simulink subsystem "Counter"  (R2022b)
settings: Solver=VariableStepAuto  StartTime=0.0  StopTime=10.0  RelTol=1e-3
model mask{counterType=Up, value=1, reset=0, cntValue=1}
  mask prompts: counterType "Counter Type"; value "Counter Value"; reset "Reset Value"
libraries: simulink x1
settings Model: Creator=MAAM  LastModifiedBy=MAAM

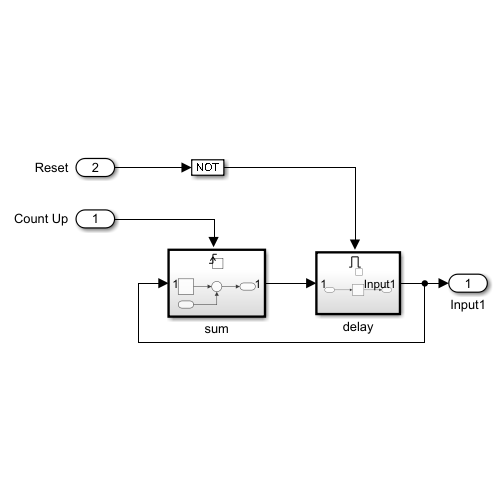
[thumbnail: Simulink's stored preview of the top-level diagram]
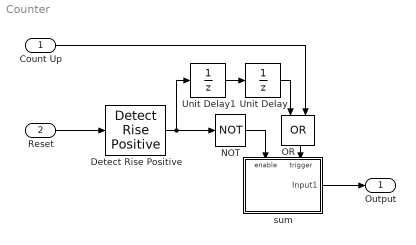
== system Counter ==
  Count Up : Inport
  Reset : Inport  Port=2
  Detect Rise Positive : simulink/Logic and Bit Operations/Detect Rise Positive  vinit=0  OutDataTypeStr=boolean
  NOT : Logic  Operator=NOT  AllPortsSameDT=off  OutDataTypeStr=boolean
  OR : Logic  Operator=OR  AllPortsSameDT=off  OutDataTypeStr=boolean
  Unit Delay : UnitDelay  SampleTime=-1  HasFrameUpgradeWarning=on
  Unit Delay1 : UnitDelay  SampleTime=-1  HasFrameUpgradeWarning=on
  sum : Subsystem
  Output : Outport
  wires:
  Count Up/1 -> OR/2
  sum/1(Input1) -> Output/1
  Unit Delay/1 -> OR/1
  OR/1 -> sum/Trigger
  Reset/1 -> Detect Rise Positive/1
  Detect Rise Positive/1 -> NOT/1, Unit Delay1/1
  Unit Delay1/1 -> Unit Delay/1
  NOT/1 -> sum/Enable

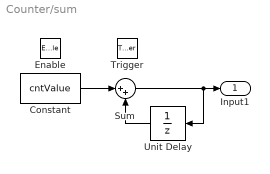
== system Counter/sum ==
  Enable : EnablePort  StatesWhenEnabling=reset
  Trigger : TriggerPort  VariantControl=(inherit)  PortDimensions=1
  Constant : Constant  Value=cntValue
  Sum : Sum  Inputs=|++
  Unit Delay : UnitDelay  InitialCondition=reset-cntValue  SampleTime=-1  HasFrameUpgradeWarning=on
  Input1 : Outport
  wires:
  Sum/1 -> Unit Delay/1, Input1/1
  Unit Delay/1 -> Sum/2
  Constant/1 -> Sum/1
